simulink model "px4_read_serial"  (R2024a)
settings: Solver=VariableStepAuto  StartTime=0.0  StopTime=100  RelTol=1e-3
libraries: uavmavlinklib x3, px4MAVLinkBridgelib x1, simulink_extras x1, aerolibanimutils x1
settings Model: Creator=user  LastModifiedBy=user

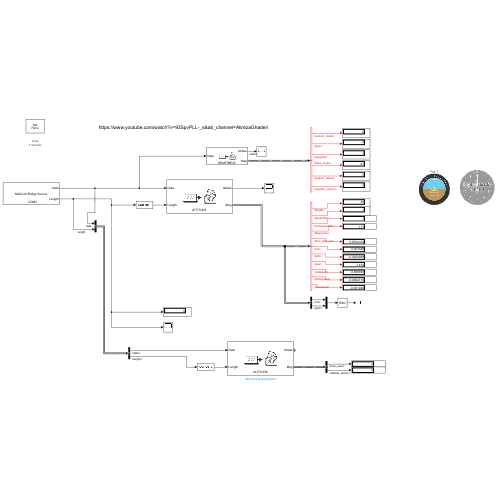
[thumbnail: Simulink's stored preview of the top-level diagram]
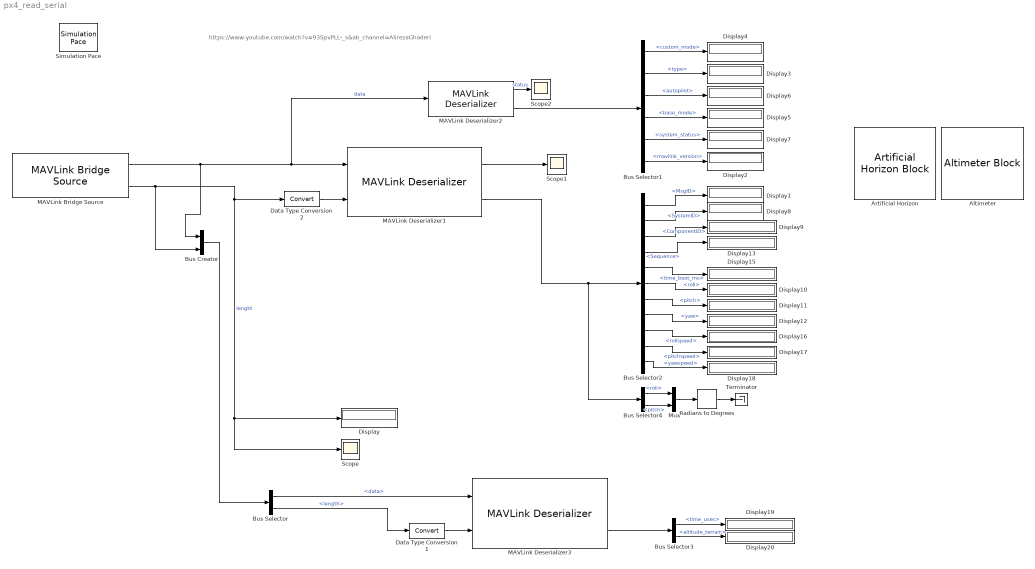
== system px4_read_serial ==
  note: https://www.youtube.com/watch?v=93SpvPLL-_s&ab_channel=AlirezaGhaderi
  Altimeter : AltimeterBlock
  Artificial Horizon : ArtificialHorizonBlock
  Bus Creator : BusCreator  Inputs=2
  Bus Selector : BusSelector  OutputSignals=data,length
  Bus Selector1 : BusSelector  OutputSignals=Payload.custom_mode,Payload.type,Payload.autopilot,Payload.base_mode,Payload.system_status,Payload.mavlink_version
  Bus Selector2 : BusSelector  OutputSignals=MsgID,SystemID,ComponentID,Sequence,Payload.time_boot_ms,Payload.roll,Payload.pitch,Payload.yaw,Payload.rollspeed,Payload.pitchspeed,Payload.yawspeed
  Bus Selector3 : BusSelector  OutputSignals=Payload.time_usec,Payload.altitude_terrain
  Bus Selector4 : BusSelector  OutputSignals=Payload.roll,Payload.pitch
  Data Type Conversion1 : DataTypeConversion  SaturateOnIntegerOverflow=off  RndMeth=Floor
  Data Type Conversion2 : DataTypeConversion  SaturateOnIntegerOverflow=off  RndMeth=Floor
  Display{,1..13,15..20} (20 alike) : Display
  MAVLink Bridge Source : px4MAVLinkBridgelib/MAVLink Bridge Source  PixhawkSerialPorttemp=COM4  PixhawkSerialPortManually=COM4  dataLength=1024  FieldTable={ 'UDP', '127.0.0.1', '14550' }  SampleTime=1/5
  MAVLink Deserializer1 : uavmavlinklib/MAVLink Deserializer  dialectSource=Select from standard MAVLink dialects  dialect=common.xml  dialectCustom=common.xml  version=2  messageType=ATTITUDE  inputDataLength=on  SystemIDFilter=off  systemID=1  ComponentIDFilter=off  componentID=1  queueMsg=off  queueMsgSize=50  dropNum=off
  MAVLink Deserializer2 : uavmavlinklib/MAVLink Deserializer  dialectSource=Select from standard MAVLink dialects  dialect=common.xml  dialectCustom=common.xml  version=2  messageType=HEARTBEAT  inputDataLength=off  SystemIDFilter=off  systemID=1  ComponentIDFilter=off  componentID=1  queueMsg=off  queueMsgSize=50  dropNum=off
  MAVLink Deserializer3 : uavmavlinklib/MAVLink Deserializer  dialectSource=Select from standard MAVLink dialects  dialect=common.xml  dialectCustom=common.xml  version=2  messageType=ALTITUDE  inputDataLength=on  SystemIDFilter=off  systemID=1  ComponentIDFilter=off  componentID=1  queueMsg=off  queueMsgSize=50  dropNum=off
  Mux : Mux  Inputs=2
  Radians to Degrees : simulink_extras/Transformations/Radians to Degrees
  Scope : Scope
  Scope1 : Scope
  Scope2 : Scope
  Simulation Pace : aerolibanimutils/Simulation Pace  SimulationPace=1  SleepMode=Auto  OutputPaceError=off  SampleTime=-1
  Terminator : Terminator
  wires:
  MAVLink Bridge Source/2 -> Scope/1, Display/1, Data Type Conversion2/1, Bus Creator/2  "length"
  Data Type Conversion2/1 -> MAVLink Deserializer1/2
  MAVLink Bridge Source/1 -> Bus Creator/1, MAVLink Deserializer2/1, MAVLink Deserializer1/1  "data"
  MAVLink Deserializer2/1 -> Scope2/1  "status"
  MAVLink Deserializer2/2 -> Bus Selector1/1
  Bus Selector1/6 -> Display2/1  "<mavlink_version>"
  Bus Selector1/2 -> Display3/1  "<type>"
  Bus Selector1/1 -> Display4/1  "<custom_mode>"
  Bus Selector1/4 -> Display5/1  "<base_mode>"
  Bus Selector1/3 -> Display6/1  "<autopilot>"
  Bus Selector1/5 -> Display7/1  "<system_status>"
  MAVLink Deserializer1/1 -> Scope1/1
  Bus Selector2/1 -> Display1/1  "<MsgID>"
  Bus Selector2/2 -> Display8/1  "<SystemID>"
  Bus Selector2/3 -> Display9/1  "<ComponentID>"
  Bus Selector2/6 -> Display10/1  "<roll>"
  Bus Selector2/7 -> Display11/1  "<pitch>"
  Bus Selector2/8 -> Display12/1  "<yaw>"
  Bus Selector2/4 -> Display13/1  "<Sequence>"
  Bus Selector2/5 -> Display15/1  "<time_boot_ms>"
  Bus Selector2/9 -> Display16/1  "<rollspeed>"
  Bus Selector2/10 -> Display17/1  "<pitchspeed>"
  Bus Selector2/11 -> Display18/1  "<yawspeed>"
  Bus Creator/1 -> Bus Selector/1
  Bus Selector/1 -> MAVLink Deserializer3/1  "<data>"
  Bus Selector/2 -> Data Type Conversion1/1  "<length>"
  MAVLink Deserializer3/2 -> Bus Selector3/1
  Bus Selector3/1 -> Display19/1  "<time_usec>"
  Bus Selector3/2 -> Display20/1  "<altitude_terrain>"
  Data Type Conversion1/1 -> MAVLink Deserializer3/2
  MAVLink Deserializer1/2 -> Bus Selector4/1, Bus Selector2/1
  Bus Selector4/1 -> Mux/1  "<roll>"
  Bus Selector4/2 -> Mux/2  "<pitch>"
  Mux/1 -> Radians to Degrees/1
  Radians to Degrees/1 -> Terminator/1
